simulink model "generic_truck"  (Simulink 10.3)
settings: Solver=ode45  StartTime=0.0  StopTime=inf  RelTol=1e-3  EnableMultiTasking=on
libraries: TruckMaker4SL x1, simulink x1
(part 3 of 3)

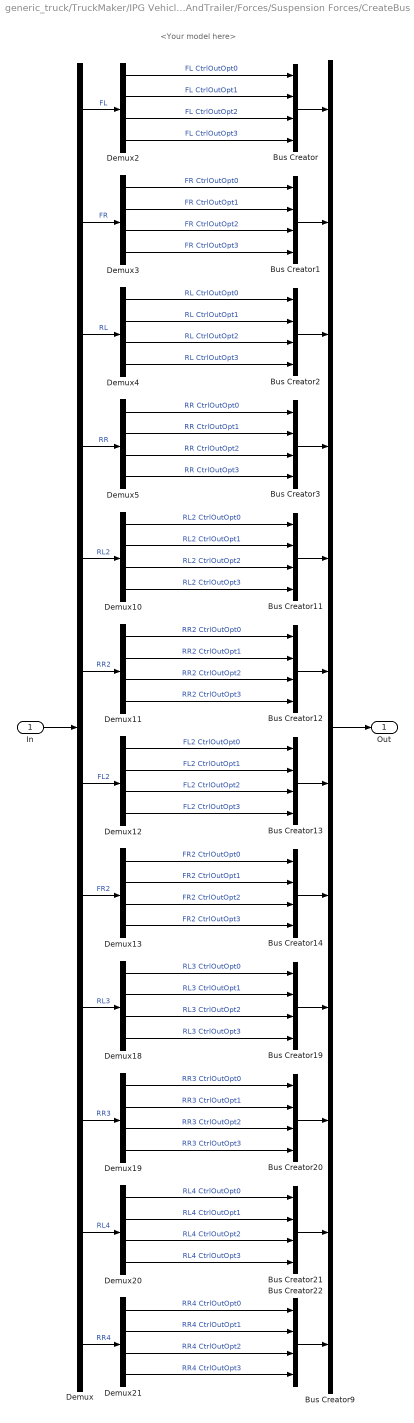
== system generic_truck/TruckMaker/IPG Vehicle/CarAndTrailer/Forces/Suspension Forces/CreateBus SpringCtrlOutOpt ==
  note: <Your model here>
  In : Inport
  Bus Creator{,1..3,11..14,19..22} (12 alike) : BusCreator  Inputs=4
  Bus Creator9 : BusCreator  Inputs=12
  Demux : Demux  Outputs=12
  Demux{2..5,10..13,18..21} (12 alike) : Demux
  Out : Outport
  wires:
  Demux/8 -> Demux13/1  "FR2"
  Demux19/1 -> Bus Creator20/1  "RR3 CtrlOutOpt0"
  Demux19/3 -> Bus Creator20/3  "RR3 CtrlOutOpt2"
  Demux18/4 -> Bus Creator19/4  "RL3 CtrlOutOpt3"
  Demux2/3 -> Bus Creator/3  "FL CtrlOutOpt2"
  Demux4/4 -> Bus Creator2/4  "RL CtrlOutOpt3"
  Demux3/2 -> Bus Creator1/2  "FR CtrlOutOpt1"
  Bus Creator11/1 -> Bus Creator9/5
  Demux2/4 -> Bus Creator/4  "FL CtrlOutOpt3"
  Demux/9 -> Demux18/1  "RL3"
  Demux10/3 -> Bus Creator11/3  "RL2 CtrlOutOpt2"
  Demux2/1 -> Bus Creator/1  "FL CtrlOutOpt0"
  Demux13/4 -> Bus Creator14/4  "FR2 CtrlOutOpt3"
  Demux19/4 -> Bus Creator20/4  "RR3 CtrlOutOpt3"
  Bus Creator1/1 -> Bus Creator9/2
  Bus Creator14/1 -> Bus Creator9/8
  Demux4/3 -> Bus Creator2/3  "RL CtrlOutOpt2"
  Demux2/2 -> Bus Creator/2  "FL CtrlOutOpt1"
  Demux5/1 -> Bus Creator3/1  "RR CtrlOutOpt0"
  Demux18/3 -> Bus Creator19/3  "RL3 CtrlOutOpt2"
  Demux12/1 -> Bus Creator13/1  "FL2 CtrlOutOpt0"
  Demux12/3 -> Bus Creator13/3  "FL2 CtrlOutOpt2"
  Bus Creator19/1 -> Bus Creator9/9
  Demux4/1 -> Bus Creator2/1  "RL CtrlOutOpt0"
  Demux10/1 -> Bus Creator11/1  "RL2 CtrlOutOpt0"
  Bus Creator/1 -> Bus Creator9/1
  Demux11/1 -> Bus Creator12/1  "RR2 CtrlOutOpt0"
  Demux20/1 -> Bus Creator21/1  "RL4 CtrlOutOpt0"
  Demux10/4 -> Bus Creator11/4  "RL2 CtrlOutOpt3"
  Bus Creator12/1 -> Bus Creator9/6
  Demux12/2 -> Bus Creator13/2  "FL2 CtrlOutOpt1"
  Demux11/3 -> Bus Creator12/3  "RR2 CtrlOutOpt2"
  Demux3/4 -> Bus Creator1/4  "FR CtrlOutOpt3"
  Demux18/2 -> Bus Creator19/2  "RL3 CtrlOutOpt1"
  Demux5/3 -> Bus Creator3/3  "RR CtrlOutOpt2"
  Demux19/2 -> Bus Creator20/2  "RR3 CtrlOutOpt1"
  Bus Creator20/1 -> Bus Creator9/10
  Demux20/2 -> Bus Creator21/2  "RL4 CtrlOutOpt1"
  Demux/7 -> Demux12/1  "FL2"
  Bus Creator2/1 -> Bus Creator9/3
  Demux/4 -> Demux5/1  "RR"
  Demux/1 -> Demux2/1  "FL"
  Demux20/4 -> Bus Creator21/4  "RL4 CtrlOutOpt3"
  Demux13/1 -> Bus Creator14/1  "FR2 CtrlOutOpt0"
  Demux/3 -> Demux4/1  "RL"
  Demux20/3 -> Bus Creator21/3  "RL4 CtrlOutOpt2"
  Demux3/1 -> Bus Creator1/1  "FR CtrlOutOpt0"
  Demux21/4 -> Bus Creator22/4  "RR4 CtrlOutOpt3"
  Demux11/4 -> Bus Creator12/4  "RR2 CtrlOutOpt3"
  Demux3/3 -> Bus Creator1/3  "FR CtrlOutOpt2"
  Demux18/1 -> Bus Creator19/1  "RL3 CtrlOutOpt0"
  Demux/10 -> Demux19/1  "RR3"
  Demux10/2 -> Bus Creator11/2  "RL2 CtrlOutOpt1"
  Demux12/4 -> Bus Creator13/4  "FL2 CtrlOutOpt3"
  Demux13/3 -> Bus Creator14/3  "FR2 CtrlOutOpt2"
  Demux4/2 -> Bus Creator2/2  "RL CtrlOutOpt1"
  Demux21/2 -> Bus Creator22/2  "RR4 CtrlOutOpt1"
  Demux5/2 -> Bus Creator3/2  "RR CtrlOutOpt1"
  Bus Creator3/1 -> Bus Creator9/4
  Demux21/3 -> Bus Creator22/3  "RR4 CtrlOutOpt2"
  Demux21/1 -> Bus Creator22/1  "RR4 CtrlOutOpt0"
  Demux/6 -> Demux11/1  "RR2"
  Demux/2 -> Demux3/1  "FR"
  Demux11/2 -> Bus Creator12/2  "RR2 CtrlOutOpt1"
  Demux13/2 -> Bus Creator14/2  "FR2 CtrlOutOpt1"
  Demux/5 -> Demux10/1  "RL2"
  Bus Creator13/1 -> Bus Creator9/7
  Demux5/4 -> Bus Creator3/4  "RR CtrlOutOpt3"
  In/1 -> Demux/1
  Bus Creator9/1 -> Out/1
  Demux/11 -> Demux20/1  "RL4"
  Bus Creator21/1 -> Bus Creator9/11
  Demux/12 -> Demux21/1  "RR4"
  Bus Creator22/1 -> Bus Creator9/12

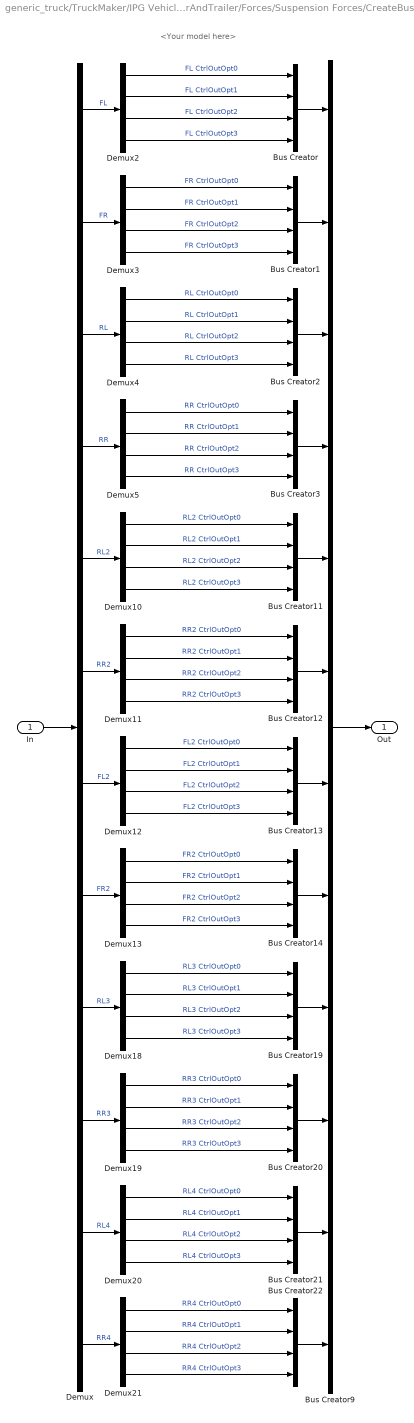
== system generic_truck/TruckMaker/IPG Vehicle/CarAndTrailer/Forces/Suspension Forces/CreateBus StabiCtrlOutOpt ==
  note: <Your model here>
  In : Inport
  Bus Creator{,1..3,11..14,19..22} (12 alike) : BusCreator  Inputs=4
  Bus Creator9 : BusCreator  Inputs=12
  Demux : Demux  Outputs=12
  Demux{2..5,10..13,18..21} (12 alike) : Demux
  Out : Outport
  wires:
  Demux/8 -> Demux13/1  "FR2"
  Demux19/1 -> Bus Creator20/1  "RR3 CtrlOutOpt0"
  Demux19/3 -> Bus Creator20/3  "RR3 CtrlOutOpt2"
  Demux18/4 -> Bus Creator19/4  "RL3 CtrlOutOpt3"
  Demux2/3 -> Bus Creator/3  "FL CtrlOutOpt2"
  Demux4/4 -> Bus Creator2/4  "RL CtrlOutOpt3"
  Demux3/2 -> Bus Creator1/2  "FR CtrlOutOpt1"
  Bus Creator11/1 -> Bus Creator9/5
  Demux2/4 -> Bus Creator/4  "FL CtrlOutOpt3"
  Demux/9 -> Demux18/1  "RL3"
  Demux10/3 -> Bus Creator11/3  "RL2 CtrlOutOpt2"
  Demux2/1 -> Bus Creator/1  "FL CtrlOutOpt0"
  Demux13/4 -> Bus Creator14/4  "FR2 CtrlOutOpt3"
  Demux19/4 -> Bus Creator20/4  "RR3 CtrlOutOpt3"
  Bus Creator1/1 -> Bus Creator9/2
  Bus Creator14/1 -> Bus Creator9/8
  Demux4/3 -> Bus Creator2/3  "RL CtrlOutOpt2"
  Demux2/2 -> Bus Creator/2  "FL CtrlOutOpt1"
  Demux5/1 -> Bus Creator3/1  "RR CtrlOutOpt0"
  Demux18/3 -> Bus Creator19/3  "RL3 CtrlOutOpt2"
  Demux12/1 -> Bus Creator13/1  "FL2 CtrlOutOpt0"
  Demux12/3 -> Bus Creator13/3  "FL2 CtrlOutOpt2"
  Bus Creator19/1 -> Bus Creator9/9
  Demux4/1 -> Bus Creator2/1  "RL CtrlOutOpt0"
  Demux10/1 -> Bus Creator11/1  "RL2 CtrlOutOpt0"
  Bus Creator/1 -> Bus Creator9/1
  Demux11/1 -> Bus Creator12/1  "RR2 CtrlOutOpt0"
  Demux20/1 -> Bus Creator21/1  "RL4 CtrlOutOpt0"
  Demux10/4 -> Bus Creator11/4  "RL2 CtrlOutOpt3"
  Bus Creator12/1 -> Bus Creator9/6
  Demux12/2 -> Bus Creator13/2  "FL2 CtrlOutOpt1"
  Demux11/3 -> Bus Creator12/3  "RR2 CtrlOutOpt2"
  Demux3/4 -> Bus Creator1/4  "FR CtrlOutOpt3"
  Demux18/2 -> Bus Creator19/2  "RL3 CtrlOutOpt1"
  Demux5/3 -> Bus Creator3/3  "RR CtrlOutOpt2"
  Demux19/2 -> Bus Creator20/2  "RR3 CtrlOutOpt1"
  Bus Creator20/1 -> Bus Creator9/10
  Demux20/2 -> Bus Creator21/2  "RL4 CtrlOutOpt1"
  Demux/7 -> Demux12/1  "FL2"
  Bus Creator2/1 -> Bus Creator9/3
  Demux/4 -> Demux5/1  "RR"
  Demux/1 -> Demux2/1  "FL"
  Demux20/4 -> Bus Creator21/4  "RL4 CtrlOutOpt3"
  Demux13/1 -> Bus Creator14/1  "FR2 CtrlOutOpt0"
  Demux/3 -> Demux4/1  "RL"
  Demux20/3 -> Bus Creator21/3  "RL4 CtrlOutOpt2"
  Demux3/1 -> Bus Creator1/1  "FR CtrlOutOpt0"
  Demux21/4 -> Bus Creator22/4  "RR4 CtrlOutOpt3"
  Demux11/4 -> Bus Creator12/4  "RR2 CtrlOutOpt3"
  Demux3/3 -> Bus Creator1/3  "FR CtrlOutOpt2"
  Demux18/1 -> Bus Creator19/1  "RL3 CtrlOutOpt0"
  Demux/10 -> Demux19/1  "RR3"
  Demux10/2 -> Bus Creator11/2  "RL2 CtrlOutOpt1"
  Demux12/4 -> Bus Creator13/4  "FL2 CtrlOutOpt3"
  Demux13/3 -> Bus Creator14/3  "FR2 CtrlOutOpt2"
  Demux4/2 -> Bus Creator2/2  "RL CtrlOutOpt1"
  Demux21/2 -> Bus Creator22/2  "RR4 CtrlOutOpt1"
  Demux5/2 -> Bus Creator3/2  "RR CtrlOutOpt1"
  Bus Creator3/1 -> Bus Creator9/4
  Demux21/3 -> Bus Creator22/3  "RR4 CtrlOutOpt2"
  Demux21/1 -> Bus Creator22/1  "RR4 CtrlOutOpt0"
  Demux/6 -> Demux11/1  "RR2"
  Demux/2 -> Demux3/1  "FR"
  Demux11/2 -> Bus Creator12/2  "RR2 CtrlOutOpt1"
  Demux13/2 -> Bus Creator14/2  "FR2 CtrlOutOpt1"
  Demux/5 -> Demux10/1  "RL2"
  Bus Creator13/1 -> Bus Creator9/7
  Demux5/4 -> Bus Creator3/4  "RR CtrlOutOpt3"
  In/1 -> Demux/1
  Bus Creator9/1 -> Out/1
  Demux/11 -> Demux20/1  "RL4"
  Bus Creator21/1 -> Bus Creator9/11
  Demux/12 -> Demux21/1  "RR4"
  Bus Creator22/1 -> Bus Creator9/12

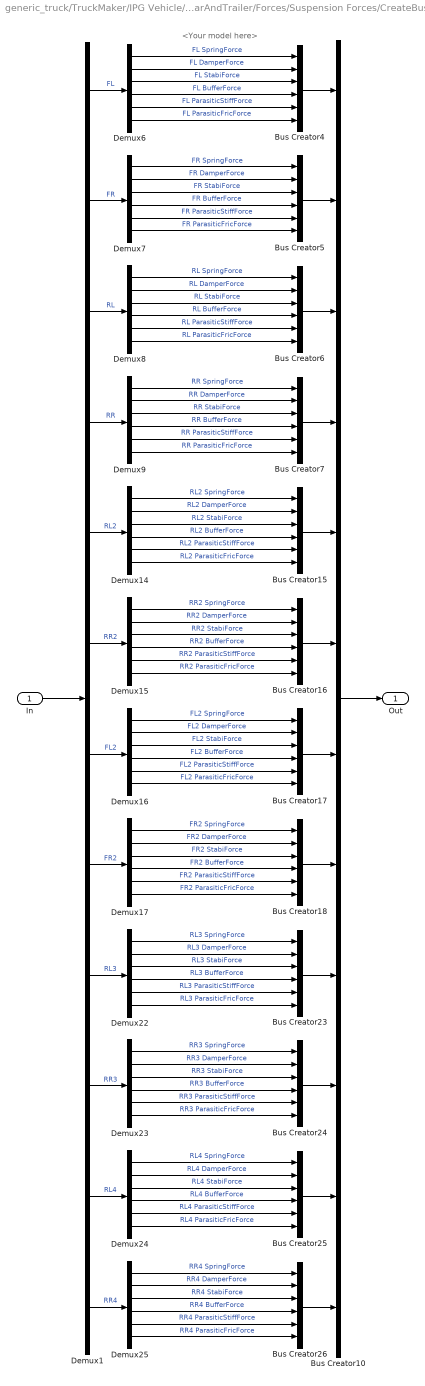
== system generic_truck/TruckMaker/IPG Vehicle/CarAndTrailer/Forces/Suspension Forces/CreateBus Suspension Forces ==
  note: <Your model here>
  In : Inport
  Bus Creator10 : BusCreator  Inputs=12
  Bus Creator{4..7,15..18,23..26} (12 alike) : BusCreator  Inputs=6
  Demux1 : Demux  Outputs=12
  Demux{6..9,14..17,22..25} (12 alike) : Demux  Outputs=6
  Out : Outport
  wires:
  Demux1/3 -> Demux8/1  "RL"
  Demux24/6 -> Bus Creator25/6  "RL4 ParasiticFricForce"
  Demux8/6 -> Bus Creator6/6  "RL ParasiticFricForce"
  Bus Creator15/1 -> Bus Creator10/5
  Demux1/11 -> Demux24/1  "RL4"
  Demux14/3 -> Bus Creator15/3  "RL2 StabiForce"
  Bus Creator7/1 -> Bus Creator10/4
  Demux16/3 -> Bus Creator17/3  "FL2 StabiForce"
  Demux1/6 -> Demux15/1  "RR2"
  Demux14/1 -> Bus Creator15/1  "RL2 SpringForce"
  Bus Creator24/1 -> Bus Creator10/10
  Demux1/10 -> Demux23/1  "RR3"
  Demux24/1 -> Bus Creator25/1  "RL4 SpringForce"
  Demux23/2 -> Bus Creator24/2  "RR3 DamperForce"
  Demux16/1 -> Bus Creator17/1  "FL2 SpringForce"
  Demux15/3 -> Bus Creator16/3  "RR2 StabiForce"
  Bus Creator17/1 -> Bus Creator10/7
  Demux15/4 -> Bus Creator16/4  "RR2 BufferForce"
  Demux17/1 -> Bus Creator18/1  "FR2 SpringForce"
  Demux6/3 -> Bus Creator4/3  "FL StabiForce"
  Demux7/4 -> Bus Creator5/4  "FR BufferForce"
  Demux14/5 -> Bus Creator15/5  "RL2 ParasiticStiffForce"
  Demux6/6 -> Bus Creator4/6  "FL ParasiticFricForce"
  Demux1/1 -> Demux6/1  "FL"
  Demux24/2 -> Bus Creator25/2  "RL4 DamperForce"
  Demux15/5 -> Bus Creator16/5  "RR2 ParasiticStiffForce"
  Demux7/3 -> Bus Creator5/3  "FR StabiForce"
  Demux9/4 -> Bus Creator7/4  "RR BufferForce"
  Demux15/6 -> Bus Creator16/6  "RR2 ParasiticFricForce"
  Demux22/3 -> Bus Creator23/3  "RL3 StabiForce"
  Demux8/2 -> Bus Creator6/2  "RL DamperForce"
  Demux1/5 -> Demux14/1  "RL2"
  Demux7/2 -> Bus Creator5/2  "FR DamperForce"
  Bus Creator6/1 -> Bus Creator10/3
  Bus Creator26/1 -> Bus Creator10/12
  Demux16/6 -> Bus Creator17/6  "FL2 ParasiticFricForce"
  Demux15/2 -> Bus Creator16/2  "RR2 DamperForce"
  Demux17/2 -> Bus Creator18/2  "FR2 DamperForce"
  Bus Creator16/1 -> Bus Creator10/6
  Demux23/4 -> Bus Creator24/4  "RR3 BufferForce"
  Demux17/6 -> Bus Creator18/6  "FR2 ParasiticFricForce"
  Demux25/5 -> Bus Creator26/5  "RR4 ParasiticStiffForce"
  Demux6/1 -> Bus Creator4/1  "FL SpringForce"
  Demux1/4 -> Demux9/1  "RR"
  Demux22/5 -> Bus Creator23/5  "RL3 ParasiticStiffForce"
  Demux9/1 -> Bus Creator7/1  "RR SpringForce"
  Demux1/2 -> Demux7/1  "FR"
  Demux1/7 -> Demux16/1  "FL2"
  Demux6/5 -> Bus Creator4/5  "FL ParasiticStiffForce"
  Bus Creator25/1 -> Bus Creator10/11
  Demux22/2 -> Bus Creator23/2  "RL3 DamperForce"
  Demux8/3 -> Bus Creator6/3  "RL StabiForce"
  Demux14/6 -> Bus Creator15/6  "RL2 ParasiticFricForce"
  Demux1/12 -> Demux25/1  "RR4"
  Bus Creator5/1 -> Bus Creator10/2
  Demux6/4 -> Bus Creator4/4  "FL BufferForce"
  Demux9/6 -> Bus Creator7/6  "RR ParasiticFricForce"
  Demux25/6 -> Bus Creator26/6  "RR4 ParasiticFricForce"
  Demux8/5 -> Bus Creator6/5  "RL ParasiticStiffForce"
  Demux8/4 -> Bus Creator6/4  "RL BufferForce"
  Demux1/9 -> Demux22/1  "RL3"
  Demux23/1 -> Bus Creator24/1  "RR3 SpringForce"
  Demux23/5 -> Bus Creator24/5  "RR3 ParasiticStiffForce"
  Demux17/5 -> Bus Creator18/5  "FR2 ParasiticStiffForce"
  Demux16/2 -> Bus Creator17/2  "FL2 DamperForce"
  Bus Creator18/1 -> Bus Creator10/8
  Demux24/4 -> Bus Creator25/4  "RL4 BufferForce"
  Demux22/6 -> Bus Creator23/6  "RL3 ParasiticFricForce"
  Demux7/5 -> Bus Creator5/5  "FR ParasiticStiffForce"
  Demux15/1 -> Bus Creator16/1  "RR2 SpringForce"
  Demux1/8 -> Demux17/1  "FR2"
  Demux25/2 -> Bus Creator26/2  "RR4 DamperForce"
  Demux14/4 -> Bus Creator15/4  "RL2 BufferForce"
  Demux14/2 -> Bus Creator15/2  "RL2 DamperForce"
  Demux9/3 -> Bus Creator7/3  "RR StabiForce"
  Demux22/1 -> Bus Creator23/1  "RL3 SpringForce"
  Demux22/4 -> Bus Creator23/4  "RL3 BufferForce"
  Demux17/4 -> Bus Creator18/4  "FR2 BufferForce"
  Demux9/2 -> Bus Creator7/2  "RR DamperForce"
  Demux16/4 -> Bus Creator17/4  "FL2 BufferForce"
  Demux25/1 -> Bus Creator26/1  "RR4 SpringForce"
  Demux25/3 -> Bus Creator26/3  "RR4 StabiForce"
  Demux23/3 -> Bus Creator24/3  "RR3 StabiForce"
  Demux7/6 -> Bus Creator5/6  "FR ParasiticFricForce"
  Bus Creator4/1 -> Bus Creator10/1
  Demux24/3 -> Bus Creator25/3  "RL4 StabiForce"
  Demux23/6 -> Bus Creator24/6  "RR3 ParasiticFricForce"
  Bus Creator23/1 -> Bus Creator10/9
  Demux7/1 -> Bus Creator5/1  "FR SpringForce"
  Demux25/4 -> Bus Creator26/4  "RR4 BufferForce"
  Demux24/5 -> Bus Creator25/5  "RL4 ParasiticStiffForce"
  Demux16/5 -> Bus Creator17/5  "FL2 ParasiticStiffForce"
  Demux17/3 -> Bus Creator18/3  "FR2 StabiForce"
  Demux6/2 -> Bus Creator4/2  "FL DamperForce"
  Demux8/1 -> Bus Creator6/1  "RL SpringForce"
  Demux9/5 -> Bus Creator7/5  "RR ParasiticStiffForce"
  In/1 -> Demux1/1
  Bus Creator10/1 -> Out/1

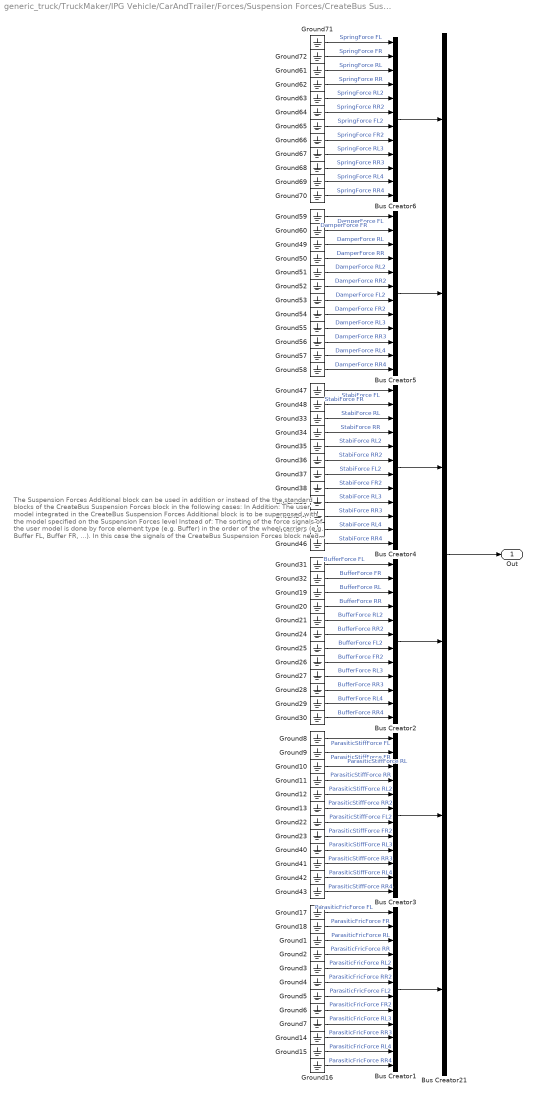
== system generic_truck/TruckMaker/IPG Vehicle/CarAndTrailer/Forces/Suspension Forces/CreateBus Suspension Forces Additional ==
  note: The Suspension Forces Additional block can be used in addition or instead of the
      | the standard blocks of the CreateBus Suspension Forces block in the following cases:
      |
      | In Addition: The user model integrated in the CreateBus Suspension Forces Additional block is to be superposed with the model specified on the Suspension Forces level
      | Instead of: The sorting of the force signals of the user model is done by force element type (e.g. Buffer) in the order of the wheel carriers (e.g. Buffer FL, Buffer FR, ...). In this case the signals of the CreateBus Suspension Forces block need to be disabled e.g. by manually connecting them to ground signals.
      |
      | ATTENTION : The forces given in the CreateBus Suspension Forces Additional block are internally added to the forces of the Suspension Forces block. If this is not desired, make sure to include a force model only in one of the two levels.
  Bus Creator{1..6} (6 alike) : BusCreator  Inputs=12
  Bus Creator21 : BusCreator  Inputs=6
  Ground{1..72} (72 alike) : Ground
  Out : Outport
  wires:
  Ground64/1 -> Bus Creator6/6  "SpringForce RR2"
  Bus Creator4/1 -> Bus Creator21/3
  Ground43/1 -> Bus Creator3/12  "ParasiticStiffForce RR4"
  Ground15/1 -> Bus Creator1/11  "ParasiticFricForce RL4"
  Ground21/1 -> Bus Creator2/5  "BufferForce RL2"
  Ground57/1 -> Bus Creator5/11  "DamperForce RL4"
  Ground14/1 -> Bus Creator1/10  "ParasiticFricForce RR3"
  Ground12/1 -> Bus Creator3/5  "ParasiticStiffForce RL2"
  Ground33/1 -> Bus Creator4/3  "StabiForce RL"
  Ground30/1 -> Bus Creator2/12  "BufferForce RR4"
  Ground13/1 -> Bus Creator3/6  "ParasiticStiffForce RR2"
  Bus Creator1/1 -> Bus Creator21/6
  Ground2/1 -> Bus Creator1/4  "ParasiticFricForce RR"
  Ground4/1 -> Bus Creator1/6  "ParasiticFricForce RR2"
  Ground27/1 -> Bus Creator2/9  "BufferForce RL3"
  Ground38/1 -> Bus Creator4/8  "StabiForce FR2"
  Ground1/1 -> Bus Creator1/3  "ParasiticFricForce RL"
  Ground36/1 -> Bus Creator4/6  "StabiForce RR2"
  Ground42/1 -> Bus Creator3/11  "ParasiticStiffForce RL4"
  Ground65/1 -> Bus Creator6/7  "SpringForce FL2"
  Ground50/1 -> Bus Creator5/4  "DamperForce RR"
  Ground67/1 -> Bus Creator6/9  "SpringForce RL3"
  Ground71/1 -> Bus Creator6/1  "SpringForce FL"
  Ground72/1 -> Bus Creator6/2  "SpringForce FR"
  Ground69/1 -> Bus Creator6/11  "SpringForce RL4"
  Ground62/1 -> Bus Creator6/4  "SpringForce RR"
  Ground51/1 -> Bus Creator5/5  "DamperForce RL2"
  Ground44/1 -> Bus Creator4/10  "StabiForce RR3"
  Ground70/1 -> Bus Creator6/12  "SpringForce RR4"
  Ground66/1 -> Bus Creator6/8  "SpringForce FR2"
  Ground40/1 -> Bus Creator3/9  "ParasiticStiffForce RL3"
  Ground16/1 -> Bus Creator1/12  "ParasiticFricForce RR4"
  Ground26/1 -> Bus Creator2/8  "BufferForce FR2"
  Ground8/1 -> Bus Creator3/1  "ParasiticStiffForce FL"
  Ground5/1 -> Bus Creator1/7  "ParasiticFricForce FL2"
  Ground29/1 -> Bus Creator2/11  "BufferForce RL4"
  Ground11/1 -> Bus Creator3/4  "ParasiticStiffForce RR"
  Ground56/1 -> Bus Creator5/10  "DamperForce RR3"
  Ground18/1 -> Bus Creator1/2  "ParasiticFricForce FR"
  Ground47/1 -> Bus Creator4/1  "StabiForce FL"
  Ground25/1 -> Bus Creator2/7  "BufferForce FL2"
  Ground32/1 -> Bus Creator2/2  "BufferForce FR"
  Ground6/1 -> Bus Creator1/8  "ParasiticFricForce FR2"
  Ground52/1 -> Bus Creator5/6  "DamperForce RR2"
  Ground24/1 -> Bus Creator2/6  "BufferForce RR2"
  Bus Creator3/1 -> Bus Creator21/5
  Ground31/1 -> Bus Creator2/1  "BufferForce FL"
  Ground68/1 -> Bus Creator6/10  "SpringForce RR3"
  Ground7/1 -> Bus Creator1/9  "ParasiticFricForce RL3"
  Ground19/1 -> Bus Creator2/3  "BufferForce RL"
  Ground9/1 -> Bus Creator3/2  "ParasiticStiffForce FR"
  Ground48/1 -> Bus Creator4/2  "StabiForce FR"
  Ground28/1 -> Bus Creator2/10  "BufferForce RR3"
  Ground61/1 -> Bus Creator6/3  "SpringForce RL"
  Ground63/1 -> Bus Creator6/5  "SpringForce RL2"
  Ground20/1 -> Bus Creator2/4  "BufferForce RR"
  Ground37/1 -> Bus Creator4/7  "StabiForce FL2"
  Bus Creator5/1 -> Bus Creator21/2
  Bus Creator21/1 -> Out/1
  Ground46/1 -> Bus Creator4/12  "StabiForce RR4"
  Ground49/1 -> Bus Creator5/3  "DamperForce RL"
  Ground35/1 -> Bus Creator4/5  "StabiForce RL2"
  Ground59/1 -> Bus Creator5/1  "DamperForce FL"
  Ground22/1 -> Bus Creator3/7  "ParasiticStiffForce FL2"
  Ground34/1 -> Bus Creator4/4  "StabiForce RR"
  Ground10/1 -> Bus Creator3/3  "ParasiticStiffForce RL"
  Ground3/1 -> Bus Creator1/5  "ParasiticFricForce RL2"
  Ground55/1 -> Bus Creator5/9  "DamperForce RL3"
  Ground60/1 -> Bus Creator5/2  "DamperForce FR"
  Ground39/1 -> Bus Creator4/9  "StabiForce RL3"
  Bus Creator2/1 -> Bus Creator21/4
  Bus Creator6/1 -> Bus Creator21/1
  Ground54/1 -> Bus Creator5/8  "DamperForce FR2"
  Ground23/1 -> Bus Creator3/8  "ParasiticStiffForce FR2"
  Ground53/1 -> Bus Creator5/7  "DamperForce FL2"
  Ground58/1 -> Bus Creator5/12  "DamperForce RR4"
  Ground17/1 -> Bus Creator1/1  "ParasiticFricForce FL"
  Ground45/1 -> Bus Creator4/11  "StabiForce RL4"
  Ground41/1 -> Bus Creator3/10  "ParasiticStiffForce RR3"

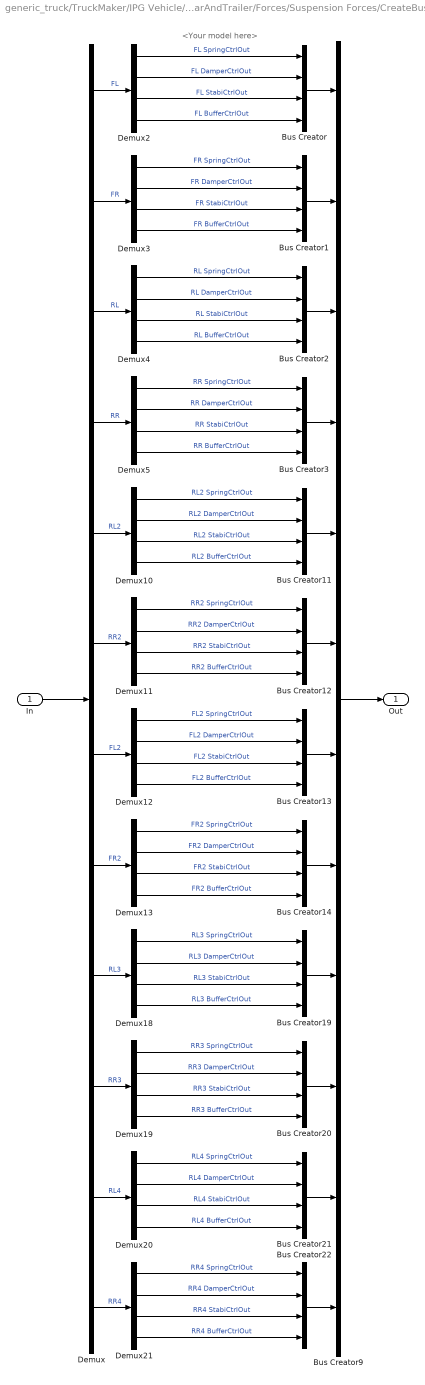
== system generic_truck/TruckMaker/IPG Vehicle/CarAndTrailer/Forces/Suspension Forces/CreateBus Suspension Forces CtrlOut ==
  note: <Your model here>
  In : Inport
  Bus Creator{,1..3,11..14,19..22} (12 alike) : BusCreator  Inputs=4
  Bus Creator9 : BusCreator  Inputs=12
  Demux : Demux  Outputs=12
  Demux{2..5,10..13,18..21} (12 alike) : Demux
  Out : Outport
  wires:
  Demux/3 -> Demux4/1  "RL"
  Demux12/3 -> Bus Creator13/3  "FL2 StabiCtrlOut"
  Demux3/1 -> Bus Creator1/1  "FR SpringCtrlOut"
  Demux3/4 -> Bus Creator1/4  "FR BufferCtrlOut"
  Demux21/2 -> Bus Creator22/2  "RR4 DamperCtrlOut"
  Demux4/3 -> Bus Creator2/3  "RL StabiCtrlOut"
  Demux18/2 -> Bus Creator19/2  "RL3 DamperCtrlOut"
  Demux19/2 -> Bus Creator20/2  "RR3 DamperCtrlOut"
  Demux13/2 -> Bus Creator14/2  "FR2 DamperCtrlOut"
  Demux10/1 -> Bus Creator11/1  "RL2 SpringCtrlOut"
  Demux20/4 -> Bus Creator21/4  "RL4 BufferCtrlOut"
  Demux/5 -> Demux10/1  "RL2"
  Demux20/3 -> Bus Creator21/3  "RL4 StabiCtrlOut"
  Bus Creator1/1 -> Bus Creator9/2
  Bus Creator19/1 -> Bus Creator9/9
  Demux10/3 -> Bus Creator11/3  "RL2 StabiCtrlOut"
  Demux5/1 -> Bus Creator3/1  "RR SpringCtrlOut"
  Demux3/2 -> Bus Creator1/2  "FR DamperCtrlOut"
  Demux13/4 -> Bus Creator14/4  "FR2 BufferCtrlOut"
  Bus Creator2/1 -> Bus Creator9/3
  Demux/12 -> Demux21/1  "RR4"
  Demux/9 -> Demux18/1  "RL3"
  Bus Creator12/1 -> Bus Creator9/6
  Bus Creator20/1 -> Bus Creator9/10
  Demux4/1 -> Bus Creator2/1  "RL SpringCtrlOut"
  Demux12/2 -> Bus Creator13/2  "FL2 DamperCtrlOut"
  Demux12/1 -> Bus Creator13/1  "FL2 SpringCtrlOut"
  Demux/4 -> Demux5/1  "RR"
  Bus Creator13/1 -> Bus Creator9/7
  Demux10/2 -> Bus Creator11/2  "RL2 DamperCtrlOut"
  Bus Creator/1 -> Bus Creator9/1
  Demux18/4 -> Bus Creator19/4  "RL3 BufferCtrlOut"
  Demux11/1 -> Bus Creator12/1  "RR2 SpringCtrlOut"
  Demux2/2 -> Bus Creator/2  "FL DamperCtrlOut"
  Demux13/3 -> Bus Creator14/3  "FR2 StabiCtrlOut"
  Demux2/4 -> Bus Creator/4  "FL BufferCtrlOut"
  Bus Creator14/1 -> Bus Creator9/8
  Demux21/3 -> Bus Creator22/3  "RR4 StabiCtrlOut"
  Demux18/3 -> Bus Creator19/3  "RL3 StabiCtrlOut"
  Demux20/2 -> Bus Creator21/2  "RL4 DamperCtrlOut"
  Demux5/4 -> Bus Creator3/4  "RR BufferCtrlOut"
  Demux/8 -> Demux13/1  "FR2"
  Demux/7 -> Demux12/1  "FL2"
  Demux20/1 -> Bus Creator21/1  "RL4 SpringCtrlOut"
  Demux21/1 -> Bus Creator22/1  "RR4 SpringCtrlOut"
  Demux13/1 -> Bus Creator14/1  "FR2 SpringCtrlOut"
  Demux5/3 -> Bus Creator3/3  "RR StabiCtrlOut"
  Demux19/3 -> Bus Creator20/3  "RR3 StabiCtrlOut"
  Demux4/2 -> Bus Creator2/2  "RL DamperCtrlOut"
  Demux/6 -> Demux11/1  "RR2"
  Demux18/1 -> Bus Creator19/1  "RL3 SpringCtrlOut"
  Demux3/3 -> Bus Creator1/3  "FR StabiCtrlOut"
  Demux/11 -> Demux20/1  "RL4"
  Bus Creator22/1 -> Bus Creator9/12
  Demux10/4 -> Bus Creator11/4  "RL2 BufferCtrlOut"
  Bus Creator11/1 -> Bus Creator9/5
  Bus Creator3/1 -> Bus Creator9/4
  Demux5/2 -> Bus Creator3/2  "RR DamperCtrlOut"
  Bus Creator21/1 -> Bus Creator9/11
  Demux/1 -> Demux2/1  "FL"
  Demux19/4 -> Bus Creator20/4  "RR3 BufferCtrlOut"
  Demux/10 -> Demux19/1  "RR3"
  Demux19/1 -> Bus Creator20/1  "RR3 SpringCtrlOut"
  Demux/2 -> Demux3/1  "FR"
  Demux2/3 -> Bus Creator/3  "FL StabiCtrlOut"
  Demux21/4 -> Bus Creator22/4  "RR4 BufferCtrlOut"
  Demux12/4 -> Bus Creator13/4  "FL2 BufferCtrlOut"
  Demux11/2 -> Bus Creator12/2  "RR2 DamperCtrlOut"
  Demux2/1 -> Bus Creator/1  "FL SpringCtrlOut"
  Demux4/4 -> Bus Creator2/4  "RL BufferCtrlOut"
  Demux11/3 -> Bus Creator12/3  "RR2 StabiCtrlOut"
  Demux11/4 -> Bus Creator12/4  "RR2 BufferCtrlOut"
  In/1 -> Demux/1
  Bus Creator9/1 -> Out/1

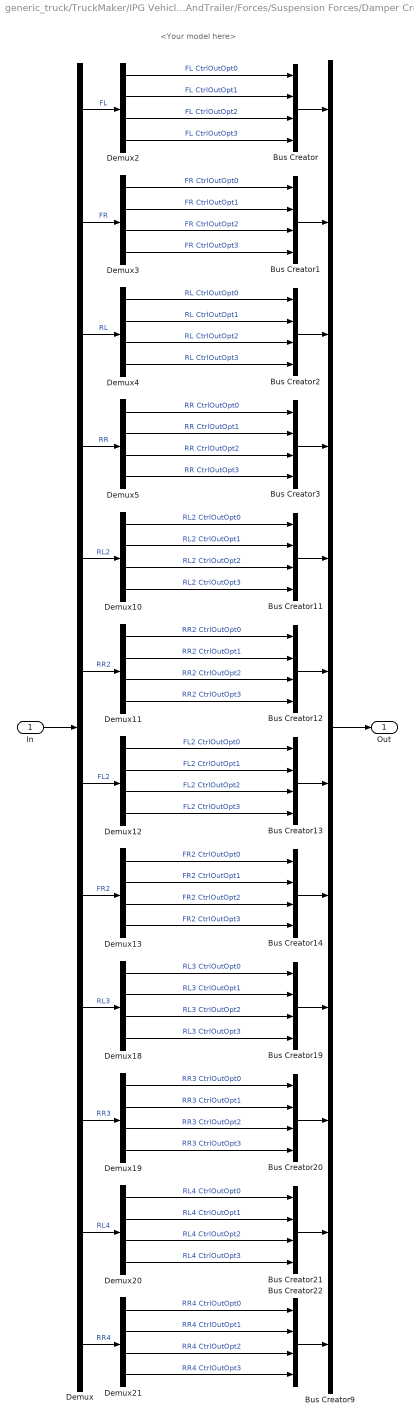
== system generic_truck/TruckMaker/IPG Vehicle/CarAndTrailer/Forces/Suspension Forces/Damper CreateBus CtrlOutOpt ==
  note: <Your model here>
  In : Inport
  Bus Creator{,1..3,11..14,19..22} (12 alike) : BusCreator  Inputs=4
  Bus Creator9 : BusCreator  Inputs=12
  Demux : Demux  Outputs=12
  Demux{2..5,10..13,18..21} (12 alike) : Demux
  Out : Outport
  wires:
  Demux/8 -> Demux13/1  "FR2"
  Demux19/1 -> Bus Creator20/1  "RR3 CtrlOutOpt0"
  Demux19/3 -> Bus Creator20/3  "RR3 CtrlOutOpt2"
  Demux18/4 -> Bus Creator19/4  "RL3 CtrlOutOpt3"
  Demux2/3 -> Bus Creator/3  "FL CtrlOutOpt2"
  Demux4/4 -> Bus Creator2/4  "RL CtrlOutOpt3"
  Demux3/2 -> Bus Creator1/2  "FR CtrlOutOpt1"
  Bus Creator11/1 -> Bus Creator9/5
  Demux2/4 -> Bus Creator/4  "FL CtrlOutOpt3"
  Demux/9 -> Demux18/1  "RL3"
  Demux10/3 -> Bus Creator11/3  "RL2 CtrlOutOpt2"
  Demux2/1 -> Bus Creator/1  "FL CtrlOutOpt0"
  Demux13/4 -> Bus Creator14/4  "FR2 CtrlOutOpt3"
  Demux19/4 -> Bus Creator20/4  "RR3 CtrlOutOpt3"
  Bus Creator1/1 -> Bus Creator9/2
  Bus Creator14/1 -> Bus Creator9/8
  Demux4/3 -> Bus Creator2/3  "RL CtrlOutOpt2"
  Demux2/2 -> Bus Creator/2  "FL CtrlOutOpt1"
  Demux5/1 -> Bus Creator3/1  "RR CtrlOutOpt0"
  Demux18/3 -> Bus Creator19/3  "RL3 CtrlOutOpt2"
  Demux12/1 -> Bus Creator13/1  "FL2 CtrlOutOpt0"
  Demux12/3 -> Bus Creator13/3  "FL2 CtrlOutOpt2"
  Bus Creator19/1 -> Bus Creator9/9
  Demux4/1 -> Bus Creator2/1  "RL CtrlOutOpt0"
  Demux10/1 -> Bus Creator11/1  "RL2 CtrlOutOpt0"
  Bus Creator/1 -> Bus Creator9/1
  Demux11/1 -> Bus Creator12/1  "RR2 CtrlOutOpt0"
  Demux20/1 -> Bus Creator21/1  "RL4 CtrlOutOpt0"
  Demux10/4 -> Bus Creator11/4  "RL2 CtrlOutOpt3"
  Bus Creator12/1 -> Bus Creator9/6
  Demux12/2 -> Bus Creator13/2  "FL2 CtrlOutOpt1"
  Demux11/3 -> Bus Creator12/3  "RR2 CtrlOutOpt2"
  Demux3/4 -> Bus Creator1/4  "FR CtrlOutOpt3"
  Demux18/2 -> Bus Creator19/2  "RL3 CtrlOutOpt1"
  Demux5/3 -> Bus Creator3/3  "RR CtrlOutOpt2"
  Demux19/2 -> Bus Creator20/2  "RR3 CtrlOutOpt1"
  Bus Creator20/1 -> Bus Creator9/10
  Demux20/2 -> Bus Creator21/2  "RL4 CtrlOutOpt1"
  Demux/7 -> Demux12/1  "FL2"
  Bus Creator2/1 -> Bus Creator9/3
  Demux/4 -> Demux5/1  "RR"
  Demux/1 -> Demux2/1  "FL"
  Demux20/4 -> Bus Creator21/4  "RL4 CtrlOutOpt3"
  Demux13/1 -> Bus Creator14/1  "FR2 CtrlOutOpt0"
  Demux/3 -> Demux4/1  "RL"
  Demux20/3 -> Bus Creator21/3  "RL4 CtrlOutOpt2"
  Demux3/1 -> Bus Creator1/1  "FR CtrlOutOpt0"
  Demux21/4 -> Bus Creator22/4  "RR4 CtrlOutOpt3"
  Demux11/4 -> Bus Creator12/4  "RR2 CtrlOutOpt3"
  Demux3/3 -> Bus Creator1/3  "FR CtrlOutOpt2"
  Demux18/1 -> Bus Creator19/1  "RL3 CtrlOutOpt0"
  Demux/10 -> Demux19/1  "RR3"
  Demux10/2 -> Bus Creator11/2  "RL2 CtrlOutOpt1"
  Demux12/4 -> Bus Creator13/4  "FL2 CtrlOutOpt3"
  Demux13/3 -> Bus Creator14/3  "FR2 CtrlOutOpt2"
  Demux4/2 -> Bus Creator2/2  "RL CtrlOutOpt1"
  Demux21/2 -> Bus Creator22/2  "RR4 CtrlOutOpt1"
  Demux5/2 -> Bus Creator3/2  "RR CtrlOutOpt1"
  Bus Creator3/1 -> Bus Creator9/4
  Demux21/3 -> Bus Creator22/3  "RR4 CtrlOutOpt2"
  Demux21/1 -> Bus Creator22/1  "RR4 CtrlOutOpt0"
  Demux/6 -> Demux11/1  "RR2"
  Demux/2 -> Demux3/1  "FR"
  Demux11/2 -> Bus Creator12/2  "RR2 CtrlOutOpt1"
  Demux13/2 -> Bus Creator14/2  "FR2 CtrlOutOpt1"
  Demux/5 -> Demux10/1  "RL2"
  Bus Creator13/1 -> Bus Creator9/7
  Demux5/4 -> Bus Creator3/4  "RR CtrlOutOpt3"
  In/1 -> Demux/1
  Bus Creator9/1 -> Out/1
  Demux/11 -> Demux20/1  "RL4"
  Bus Creator21/1 -> Bus Creator9/11
  Demux/12 -> Demux21/1  "RR4"
  Bus Creator22/1 -> Bus Creator9/12

== system generic_truck/TruckMaker/IPG Vehicle/CarAndTrailer/Forces/Suspension Forces/FrcSystem CreateBus CtrlOutOpt ==
  note: <Your model here>
  In : Inport
  Bus Creator9 : BusCreator  Inputs=192
  Demux : Demux  Outputs=192
  Out : Outport
  wires:
  In/1 -> Demux/1
  Bus Creator9/1 -> Out/1
  Demux/64 -> Bus Creator9/64  "CtrlOutOpt63"
  Demux/1 -> Bus Creator9/1  "CtrlOutOpt0"
  Demux/2 -> Bus Creator9/2  "CtrlOutOpt1"
  Demux/3 -> Bus Creator9/3  "CtrlOutOpt2"
  Demux/4 -> Bus Creator9/4  "CtrlOutOpt3"
  Demux/5 -> Bus Creator9/5  "CtrlOutOpt4"
  Demux/6 -> Bus Creator9/6  "CtrlOutOpt5"
  Demux/7 -> Bus Creator9/7  "CtrlOutOpt6"
  Demux/8 -> Bus Creator9/8  "CtrlOutOpt7"
  Demux/9 -> Bus Creator9/9  "CtrlOutOpt8"
  Demux/10 -> Bus Creator9/10  "CtrlOutOpt9"
  Demux/11 -> Bus Creator9/11  "CtrlOutOpt10"
  Demux/12 -> Bus Creator9/12  "CtrlOutOpt11"
  Demux/13 -> Bus Creator9/13  "CtrlOutOpt12"
  Demux/14 -> Bus Creator9/14  "CtrlOutOpt13"
  Demux/15 -> Bus Creator9/15  "CtrlOutOpt14"
  Demux/16 -> Bus Creator9/16  "CtrlOutOpt15"
  Demux/17 -> Bus Creator9/17  "CtrlOutOpt16"
  Demux/18 -> Bus Creator9/18  "CtrlOutOpt17"
  Demux/19 -> Bus Creator9/19  "CtrlOutOpt18"
  Demux/20 -> Bus Creator9/20  "CtrlOutOpt19"
  Demux/21 -> Bus Creator9/21  "CtrlOutOpt20"
  Demux/22 -> Bus Creator9/22  "CtrlOutOpt21"
  Demux/23 -> Bus Creator9/23  "CtrlOutOpt22"
  Demux/24 -> Bus Creator9/24  "CtrlOutOpt23"
  Demux/25 -> Bus Creator9/25  "CtrlOutOpt24"
  Demux/26 -> Bus Creator9/26  "CtrlOutOpt25"
  Demux/27 -> Bus Creator9/27  "CtrlOutOpt26"
  Demux/28 -> Bus Creator9/28  "CtrlOutOpt27"
  Demux/29 -> Bus Creator9/29  "CtrlOutOpt28"
  Demux/30 -> Bus Creator9/30  "CtrlOutOpt29"
  Demux/31 -> Bus Creator9/31  "CtrlOutOpt30"
  Demux/32 -> Bus Creator9/32  "CtrlOutOpt31"
  Demux/33 -> Bus Creator9/33  "CtrlOutOpt32"
  Demux/34 -> Bus Creator9/34  "CtrlOutOpt33"
  Demux/35 -> Bus Creator9/35  "CtrlOutOpt34"
  Demux/36 -> Bus Creator9/36  "CtrlOutOpt35"
  Demux/37 -> Bus Creator9/37  "CtrlOutOpt36"
  Demux/38 -> Bus Creator9/38  "CtrlOutOpt37"
  Demux/39 -> Bus Creator9/39  "CtrlOutOpt38"
  Demux/40 -> Bus Creator9/40  "CtrlOutOpt39"
  Demux/41 -> Bus Creator9/41  "CtrlOutOpt40"
  Demux/42 -> Bus Creator9/42  "CtrlOutOpt41"
  Demux/43 -> Bus Creator9/43  "CtrlOutOpt42"
  Demux/44 -> Bus Creator9/44  "CtrlOutOpt43"
  Demux/45 -> Bus Creator9/45  "CtrlOutOpt44"
  Demux/46 -> Bus Creator9/46  "CtrlOutOpt45"
  Demux/47 -> Bus Creator9/47  "CtrlOutOpt46"
  Demux/48 -> Bus Creator9/48  "CtrlOutOpt47"
  Demux/49 -> Bus Creator9/49  "CtrlOutOpt48"
  Demux/50 -> Bus Creator9/50  "CtrlOutOpt49"
  Demux/51 -> Bus Creator9/51  "CtrlOutOpt50"
  Demux/52 -> Bus Creator9/52  "CtrlOutOpt51"
  Demux/53 -> Bus Creator9/53  "CtrlOutOpt52"
  Demux/54 -> Bus Creator9/54  "CtrlOutOpt53"
  Demux/55 -> Bus Creator9/55  "CtrlOutOpt54"
  Demux/56 -> Bus Creator9/56  "CtrlOutOpt55"
  Demux/57 -> Bus Creator9/57  "CtrlOutOpt56"
  Demux/58 -> Bus Creator9/58  "CtrlOutOpt57"
  Demux/59 -> Bus Creator9/59  "CtrlOutOpt58"
  Demux/60 -> Bus Creator9/60  "CtrlOutOpt59"
  Demux/61 -> Bus Creator9/61  "CtrlOutOpt60"
  Demux/62 -> Bus Creator9/62  "CtrlOutOpt61"
  Demux/63 -> Bus Creator9/63  "CtrlOutOpt62"
  Demux/65 -> Bus Creator9/65  "CtrlOutOpt64"
  Demux/66 -> Bus Creator9/66  "CtrlOutOpt65"
  Demux/67 -> Bus Creator9/67  "CtrlOutOpt66"
  Demux/68 -> Bus Creator9/68  "CtrlOutOpt67"
  Demux/69 -> Bus Creator9/69  "CtrlOutOpt68"
  Demux/70 -> Bus Creator9/70  "CtrlOutOpt69"
  Demux/71 -> Bus Creator9/71  "CtrlOutOpt70"
  Demux/72 -> Bus Creator9/72  "CtrlOutOpt71"
  Demux/73 -> Bus Creator9/73  "CtrlOutOpt72"
  Demux/74 -> Bus Creator9/74  "CtrlOutOpt73"
  Demux/75 -> Bus Creator9/75  "CtrlOutOpt74"
  Demux/76 -> Bus Creator9/76  "CtrlOutOpt75"
  Demux/77 -> Bus Creator9/77  "CtrlOutOpt76"
  Demux/78 -> Bus Creator9/78  "CtrlOutOpt77"
  Demux/79 -> Bus Creator9/79  "CtrlOutOpt78"
  Demux/80 -> Bus Creator9/80  "CtrlOutOpt79"
  Demux/81 -> Bus Creator9/81  "CtrlOutOpt80"
  Demux/82 -> Bus Creator9/82  "CtrlOutOpt81"
  Demux/83 -> Bus Creator9/83  "CtrlOutOpt82"
  Demux/84 -> Bus Creator9/84  "CtrlOutOpt83"
  Demux/85 -> Bus Creator9/85  "CtrlOutOpt84"
  Demux/86 -> Bus Creator9/86  "CtrlOutOpt85"
  Demux/87 -> Bus Creator9/87  "CtrlOutOpt86"
  Demux/88 -> Bus Creator9/88  "CtrlOutOpt87"
  Demux/89 -> Bus Creator9/89  "CtrlOutOpt88"
  Demux/90 -> Bus Creator9/90  "CtrlOutOpt89"
  Demux/91 -> Bus Creator9/91  "CtrlOutOpt90"
  Demux/92 -> Bus Creator9/92  "CtrlOutOpt91"
  Demux/93 -> Bus Creator9/93  "CtrlOutOpt92"
  Demux/94 -> Bus Creator9/94  "CtrlOutOpt93"
  Demux/95 -> Bus Creator9/95  "CtrlOutOpt94"
  Demux/96 -> Bus Creator9/96  "CtrlOutOpt95"
  Demux/97 -> Bus Creator9/97  "CtrlOutOpt96"
  Demux/98 -> Bus Creator9/98  "CtrlOutOpt97"
  Demux/99 -> Bus Creator9/99  "CtrlOutOpt98"
  Demux/100 -> Bus Creator9/100  "CtrlOutOpt99"
  Demux/101 -> Bus Creator9/101  "CtrlOutOpt100"
  Demux/102 -> Bus Creator9/102  "CtrlOutOpt101"
  Demux/103 -> Bus Creator9/103  "CtrlOutOpt102"
  Demux/104 -> Bus Creator9/104  "CtrlOutOpt103"
  Demux/105 -> Bus Creator9/105  "CtrlOutOpt104"
  Demux/106 -> Bus Creator9/106  "CtrlOutOpt105"
  Demux/107 -> Bus Creator9/107  "CtrlOutOpt106"
  Demux/108 -> Bus Creator9/108  "CtrlOutOpt107"
  Demux/109 -> Bus Creator9/109  "CtrlOutOpt108"
  Demux/110 -> Bus Creator9/110  "CtrlOutOpt109"
  Demux/111 -> Bus Creator9/111  "CtrlOutOpt110"
  Demux/112 -> Bus Creator9/112  "CtrlOutOpt111"
  Demux/113 -> Bus Creator9/113  "CtrlOutOpt112"
  Demux/114 -> Bus Creator9/114  "CtrlOutOpt113"
  Demux/115 -> Bus Creator9/115  "CtrlOutOpt114"
  Demux/116 -> Bus Creator9/116  "CtrlOutOpt115"
  Demux/117 -> Bus Creator9/117  "CtrlOutOpt116"
  Demux/118 -> Bus Creator9/118  "CtrlOutOpt117"
  Demux/119 -> Bus Creator9/119  "CtrlOutOpt118"
  Demux/120 -> Bus Creator9/120  "CtrlOutOpt119"
  Demux/121 -> Bus Creator9/121  "CtrlOutOpt120"
  Demux/122 -> Bus Creator9/122  "CtrlOutOpt121"
  Demux/123 -> Bus Creator9/123  "CtrlOutOpt122"
  Demux/124 -> Bus Creator9/124  "CtrlOutOpt123"
  Demux/125 -> Bus Creator9/125  "CtrlOutOpt124"
  Demux/126 -> Bus Creator9/126  "CtrlOutOpt125"
  Demux/127 -> Bus Creator9/127  "CtrlOutOpt126"
  Demux/128 -> Bus Creator9/128  "CtrlOutOpt127"
  Demux/129 -> Bus Creator9/129  "CtrlOutOpt128"
  Demux/130 -> Bus Creator9/130  "CtrlOutOpt129"
  Demux/131 -> Bus Creator9/131  "CtrlOutOpt130"
  Demux/132 -> Bus Creator9/132  "CtrlOutOpt131"
  Demux/133 -> Bus Creator9/133  "CtrlOutOpt132"
  Demux/134 -> Bus Creator9/134  "CtrlOutOpt133"
  Demux/135 -> Bus Creator9/135  "CtrlOutOpt134"
  Demux/136 -> Bus Creator9/136  "CtrlOutOpt135"
  Demux/137 -> Bus Creator9/137  "CtrlOutOpt136"
  Demux/138 -> Bus Creator9/138  "CtrlOutOpt137"
  Demux/139 -> Bus Creator9/139  "CtrlOutOpt138"
  Demux/140 -> Bus Creator9/140  "CtrlOutOpt139"
  Demux/141 -> Bus Creator9/141  "CtrlOutOpt140"
  Demux/142 -> Bus Creator9/142  "CtrlOutOpt141"
  Demux/143 -> Bus Creator9/143  "CtrlOutOpt142"
  Demux/144 -> Bus Creator9/144  "CtrlOutOpt143"
  Demux/145 -> Bus Creator9/145  "CtrlOutOpt144"
  Demux/146 -> Bus Creator9/146  "CtrlOutOpt145"
  Demux/147 -> Bus Creator9/147  "CtrlOutOpt146"
  Demux/148 -> Bus Creator9/148  "CtrlOutOpt147"
  Demux/149 -> Bus Creator9/149  "CtrlOutOpt148"
  Demux/150 -> Bus Creator9/150  "CtrlOutOpt149"
  Demux/151 -> Bus Creator9/151  "CtrlOutOpt150"
  Demux/152 -> Bus Creator9/152  "CtrlOutOpt151"
  Demux/153 -> Bus Creator9/153  "CtrlOutOpt152"
  Demux/154 -> Bus Creator9/154  "CtrlOutOpt153"
  Demux/155 -> Bus Creator9/155  "CtrlOutOpt154"
  Demux/156 -> Bus Creator9/156  "CtrlOutOpt155"
  Demux/157 -> Bus Creator9/157  "CtrlOutOpt156"
  Demux/158 -> Bus Creator9/158  "CtrlOutOpt157"
  Demux/159 -> Bus Creator9/159  "CtrlOutOpt158"
  Demux/160 -> Bus Creator9/160  "CtrlOutOpt159"
  Demux/161 -> Bus Creator9/161  "CtrlOutOpt160"
  Demux/162 -> Bus Creator9/162  "CtrlOutOpt161"
  Demux/163 -> Bus Creator9/163  "CtrlOutOpt162"
  Demux/164 -> Bus Creator9/164  "CtrlOutOpt163"
  Demux/165 -> Bus Creator9/165  "CtrlOutOpt164"
  Demux/166 -> Bus Creator9/166  "CtrlOutOpt165"
  Demux/167 -> Bus Creator9/167  "CtrlOutOpt166"
  Demux/168 -> Bus Creator9/168  "CtrlOutOpt167"
  Demux/169 -> Bus Creator9/169  "CtrlOutOpt168"
  Demux/170 -> Bus Creator9/170  "CtrlOutOpt169"
  Demux/171 -> Bus Creator9/171  "CtrlOutOpt170"
  Demux/172 -> Bus Creator9/172  "CtrlOutOpt171"
  Demux/173 -> Bus Creator9/173  "CtrlOutOpt172"
  Demux/174 -> Bus Creator9/174  "CtrlOutOpt173"
  Demux/175 -> Bus Creator9/175  "CtrlOutOpt174"
  Demux/176 -> Bus Creator9/176  "CtrlOutOpt175"
  Demux/177 -> Bus Creator9/177  "CtrlOutOpt176"
  Demux/178 -> Bus Creator9/178  "CtrlOutOpt177"
  Demux/179 -> Bus Creator9/179  "CtrlOutOpt178"
  Demux/180 -> Bus Creator9/180  "CtrlOutOpt179"
  Demux/181 -> Bus Creator9/181  "CtrlOutOpt180"
  Demux/182 -> Bus Creator9/182  "CtrlOutOpt181"
  Demux/183 -> Bus Creator9/183  "CtrlOutOpt182"
  Demux/184 -> Bus Creator9/184  "CtrlOutOpt183"
  Demux/185 -> Bus Creator9/185  "CtrlOutOpt184"
  Demux/186 -> Bus Creator9/186  "CtrlOutOpt185"
  Demux/187 -> Bus Creator9/187  "CtrlOutOpt186"
  Demux/188 -> Bus Creator9/188  "CtrlOutOpt187"
  Demux/189 -> Bus Creator9/189  "CtrlOutOpt188"
  Demux/190 -> Bus Creator9/190  "CtrlOutOpt189"
  Demux/191 -> Bus Creator9/191  "CtrlOutOpt190"
  Demux/192 -> Bus Creator9/192  "CtrlOutOpt191"

== system generic_truck/TruckMaker/IPG Vehicle/CarAndTrailer/Forces/Suspension Forces/Spring CreateBus CtrlOutOpt ==
  note: <Your model here>
  In : Inport
  Bus Creator{,1..3,11..14,19..22} (12 alike) : BusCreator  Inputs=4
  Bus Creator9 : BusCreator  Inputs=12
  Demux : Demux  Outputs=12
  Demux{2..5,10..13,18..21} (12 alike) : Demux
  Out : Outport
  wires:
  Demux/8 -> Demux13/1  "FR2"
  Demux19/1 -> Bus Creator20/1  "RR3 CtrlOutOpt0"
  Demux19/3 -> Bus Creator20/3  "RR3 CtrlOutOpt2"
  Demux18/4 -> Bus Creator19/4  "RL3 CtrlOutOpt3"
  Demux2/3 -> Bus Creator/3  "FL CtrlOutOpt2"
  Demux4/4 -> Bus Creator2/4  "RL CtrlOutOpt3"
  Demux3/2 -> Bus Creator1/2  "FR CtrlOutOpt1"
  Bus Creator11/1 -> Bus Creator9/5
  Demux2/4 -> Bus Creator/4  "FL CtrlOutOpt3"
  Demux/9 -> Demux18/1  "RL3"
  Demux10/3 -> Bus Creator11/3  "RL2 CtrlOutOpt2"
  Demux2/1 -> Bus Creator/1  "FL CtrlOutOpt0"
  Demux13/4 -> Bus Creator14/4  "FR2 CtrlOutOpt3"
  Demux19/4 -> Bus Creator20/4  "RR3 CtrlOutOpt3"
  Bus Creator1/1 -> Bus Creator9/2
  Bus Creator14/1 -> Bus Creator9/8
  Demux4/3 -> Bus Creator2/3  "RL CtrlOutOpt2"
  Demux2/2 -> Bus Creator/2  "FL CtrlOutOpt1"
  Demux5/1 -> Bus Creator3/1  "RR CtrlOutOpt0"
  Demux18/3 -> Bus Creator19/3  "RL3 CtrlOutOpt2"
  Demux12/1 -> Bus Creator13/1  "FL2 CtrlOutOpt0"
  Demux12/3 -> Bus Creator13/3  "FL2 CtrlOutOpt2"
  Bus Creator19/1 -> Bus Creator9/9
  Demux4/1 -> Bus Creator2/1  "RL CtrlOutOpt0"
  Demux10/1 -> Bus Creator11/1  "RL2 CtrlOutOpt0"
  Bus Creator/1 -> Bus Creator9/1
  Demux11/1 -> Bus Creator12/1  "RR2 CtrlOutOpt0"
  Demux20/1 -> Bus Creator21/1  "RL4 CtrlOutOpt0"
  Demux10/4 -> Bus Creator11/4  "RL2 CtrlOutOpt3"
  Bus Creator12/1 -> Bus Creator9/6
  Demux12/2 -> Bus Creator13/2  "FL2 CtrlOutOpt1"
  Demux11/3 -> Bus Creator12/3  "RR2 CtrlOutOpt2"
  Demux3/4 -> Bus Creator1/4  "FR CtrlOutOpt3"
  Demux18/2 -> Bus Creator19/2  "RL3 CtrlOutOpt1"
  Demux5/3 -> Bus Creator3/3  "RR CtrlOutOpt2"
  Demux19/2 -> Bus Creator20/2  "RR3 CtrlOutOpt1"
  Bus Creator20/1 -> Bus Creator9/10
  Demux20/2 -> Bus Creator21/2  "RL4 CtrlOutOpt1"
  Demux/7 -> Demux12/1  "FL2"
  Bus Creator2/1 -> Bus Creator9/3
  Demux/4 -> Demux5/1  "RR"
  Demux/1 -> Demux2/1  "FL"
  Demux20/4 -> Bus Creator21/4  "RL4 CtrlOutOpt3"
  Demux13/1 -> Bus Creator14/1  "FR2 CtrlOutOpt0"
  Demux/3 -> Demux4/1  "RL"
  Demux20/3 -> Bus Creator21/3  "RL4 CtrlOutOpt2"
  Demux3/1 -> Bus Creator1/1  "FR CtrlOutOpt0"
  Demux21/4 -> Bus Creator22/4  "RR4 CtrlOutOpt3"
  Demux11/4 -> Bus Creator12/4  "RR2 CtrlOutOpt3"
  Demux3/3 -> Bus Creator1/3  "FR CtrlOutOpt2"
  Demux18/1 -> Bus Creator19/1  "RL3 CtrlOutOpt0"
  Demux/10 -> Demux19/1  "RR3"
  Demux10/2 -> Bus Creator11/2  "RL2 CtrlOutOpt1"
  Demux12/4 -> Bus Creator13/4  "FL2 CtrlOutOpt3"
  Demux13/3 -> Bus Creator14/3  "FR2 CtrlOutOpt2"
  Demux4/2 -> Bus Creator2/2  "RL CtrlOutOpt1"
  Demux21/2 -> Bus Creator22/2  "RR4 CtrlOutOpt1"
  Demux5/2 -> Bus Creator3/2  "RR CtrlOutOpt1"
  Bus Creator3/1 -> Bus Creator9/4
  Demux21/3 -> Bus Creator22/3  "RR4 CtrlOutOpt2"
  Demux21/1 -> Bus Creator22/1  "RR4 CtrlOutOpt0"
  Demux/6 -> Demux11/1  "RR2"
  Demux/2 -> Demux3/1  "FR"
  Demux11/2 -> Bus Creator12/2  "RR2 CtrlOutOpt1"
  Demux13/2 -> Bus Creator14/2  "FR2 CtrlOutOpt1"
  Demux/5 -> Demux10/1  "RL2"
  Bus Creator13/1 -> Bus Creator9/7
  Demux5/4 -> Bus Creator3/4  "RR CtrlOutOpt3"
  In/1 -> Demux/1
  Bus Creator9/1 -> Out/1
  Demux/11 -> Demux20/1  "RL4"
  Bus Creator21/1 -> Bus Creator9/11
  Demux/12 -> Demux21/1  "RR4"
  Bus Creator22/1 -> Bus Creator9/12

== system generic_truck/TruckMaker/IPG Vehicle/CarAndTrailer/Forces/Suspension Forces/Stabi CreateBus CtrlOutOpt ==
  note: <Your model here>
  In : Inport
  Bus Creator{,1..3,11..14,19..22} (12 alike) : BusCreator  Inputs=4
  Bus Creator9 : BusCreator  Inputs=12
  Demux : Demux  Outputs=12
  Demux{2..5,10..13,18..21} (12 alike) : Demux
  Out : Outport
  wires:
  Demux/8 -> Demux13/1  "FR2"
  Demux19/1 -> Bus Creator20/1  "RR3 CtrlOutOpt0"
  Demux19/3 -> Bus Creator20/3  "RR3 CtrlOutOpt2"
  Demux18/4 -> Bus Creator19/4  "RL3 CtrlOutOpt3"
  Demux2/3 -> Bus Creator/3  "FL CtrlOutOpt2"
  Demux4/4 -> Bus Creator2/4  "RL CtrlOutOpt3"
  Demux3/2 -> Bus Creator1/2  "FR CtrlOutOpt1"
  Bus Creator11/1 -> Bus Creator9/5
  Demux2/4 -> Bus Creator/4  "FL CtrlOutOpt3"
  Demux/9 -> Demux18/1  "RL3"
  Demux10/3 -> Bus Creator11/3  "RL2 CtrlOutOpt2"
  Demux2/1 -> Bus Creator/1  "FL CtrlOutOpt0"
  Demux13/4 -> Bus Creator14/4  "FR2 CtrlOutOpt3"
  Demux19/4 -> Bus Creator20/4  "RR3 CtrlOutOpt3"
  Bus Creator1/1 -> Bus Creator9/2
  Bus Creator14/1 -> Bus Creator9/8
  Demux4/3 -> Bus Creator2/3  "RL CtrlOutOpt2"
  Demux2/2 -> Bus Creator/2  "FL CtrlOutOpt1"
  Demux5/1 -> Bus Creator3/1  "RR CtrlOutOpt0"
  Demux18/3 -> Bus Creator19/3  "RL3 CtrlOutOpt2"
  Demux12/1 -> Bus Creator13/1  "FL2 CtrlOutOpt0"
  Demux12/3 -> Bus Creator13/3  "FL2 CtrlOutOpt2"
  Bus Creator19/1 -> Bus Creator9/9
  Demux4/1 -> Bus Creator2/1  "RL CtrlOutOpt0"
  Demux10/1 -> Bus Creator11/1  "RL2 CtrlOutOpt0"
  Bus Creator/1 -> Bus Creator9/1
  Demux11/1 -> Bus Creator12/1  "RR2 CtrlOutOpt0"
  Demux20/1 -> Bus Creator21/1  "RL4 CtrlOutOpt0"
  Demux10/4 -> Bus Creator11/4  "RL2 CtrlOutOpt3"
  Bus Creator12/1 -> Bus Creator9/6
  Demux12/2 -> Bus Creator13/2  "FL2 CtrlOutOpt1"
  Demux11/3 -> Bus Creator12/3  "RR2 CtrlOutOpt2"
  Demux3/4 -> Bus Creator1/4  "FR CtrlOutOpt3"
  Demux18/2 -> Bus Creator19/2  "RL3 CtrlOutOpt1"
  Demux5/3 -> Bus Creator3/3  "RR CtrlOutOpt2"
  Demux19/2 -> Bus Creator20/2  "RR3 CtrlOutOpt1"
  Bus Creator20/1 -> Bus Creator9/10
  Demux20/2 -> Bus Creator21/2  "RL4 CtrlOutOpt1"
  Demux/7 -> Demux12/1  "FL2"
  Bus Creator2/1 -> Bus Creator9/3
  Demux/4 -> Demux5/1  "RR"
  Demux/1 -> Demux2/1  "FL"
  Demux20/4 -> Bus Creator21/4  "RL4 CtrlOutOpt3"
  Demux13/1 -> Bus Creator14/1  "FR2 CtrlOutOpt0"
  Demux/3 -> Demux4/1  "RL"
  Demux20/3 -> Bus Creator21/3  "RL4 CtrlOutOpt2"
  Demux3/1 -> Bus Creator1/1  "FR CtrlOutOpt0"
  Demux21/4 -> Bus Creator22/4  "RR4 CtrlOutOpt3"
  Demux11/4 -> Bus Creator12/4  "RR2 CtrlOutOpt3"
  Demux3/3 -> Bus Creator1/3  "FR CtrlOutOpt2"
  Demux18/1 -> Bus Creator19/1  "RL3 CtrlOutOpt0"
  Demux/10 -> Demux19/1  "RR3"
  Demux10/2 -> Bus Creator11/2  "RL2 CtrlOutOpt1"
  Demux12/4 -> Bus Creator13/4  "FL2 CtrlOutOpt3"
  Demux13/3 -> Bus Creator14/3  "FR2 CtrlOutOpt2"
  Demux4/2 -> Bus Creator2/2  "RL CtrlOutOpt1"
  Demux21/2 -> Bus Creator22/2  "RR4 CtrlOutOpt1"
  Demux5/2 -> Bus Creator3/2  "RR CtrlOutOpt1"
  Bus Creator3/1 -> Bus Creator9/4
  Demux21/3 -> Bus Creator22/3  "RR4 CtrlOutOpt2"
  Demux21/1 -> Bus Creator22/1  "RR4 CtrlOutOpt0"
  Demux/6 -> Demux11/1  "RR2"
  Demux/2 -> Demux3/1  "FR"
  Demux11/2 -> Bus Creator12/2  "RR2 CtrlOutOpt1"
  Demux13/2 -> Bus Creator14/2  "FR2 CtrlOutOpt1"
  Demux/5 -> Demux10/1  "RL2"
  Bus Creator13/1 -> Bus Creator9/7
  Demux5/4 -> Bus Creator3/4  "RR CtrlOutOpt3"
  In/1 -> Demux/1
  Bus Creator9/1 -> Out/1
  Demux/11 -> Demux20/1  "RL4"
  Bus Creator21/1 -> Bus Creator9/11
  Demux/12 -> Demux21/1  "RR4"
  Bus Creator22/1 -> Bus Creator9/12
